simulink library "csc_thm_thermal_system_sim_lib"  (R2014b)
settings: Solver=ode45  StartTime=0.0  StopTime=10.0  RelTol=1e-3
values from neighbouring files (symbols this model uses):
  thm_model_update_counter = round(thm_time_step/sim_time_step_size)    [csc_thm_thermal_system_sim_prep.m]
undefined symbols (not defined in the file or in its folder): stm_time_step
libraries: util_info_lib x1, csc_stm_simplified_temperature_model_collection_lib x1, simulink x1
settings Model: Creator=escrane  LastModifiedBy=mstewart

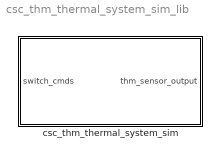
== system csc_thm_thermal_system_sim_lib ==
  csc_thm_thermal_system_sim : Subsystem  SystemSampleTime=stm_time_step

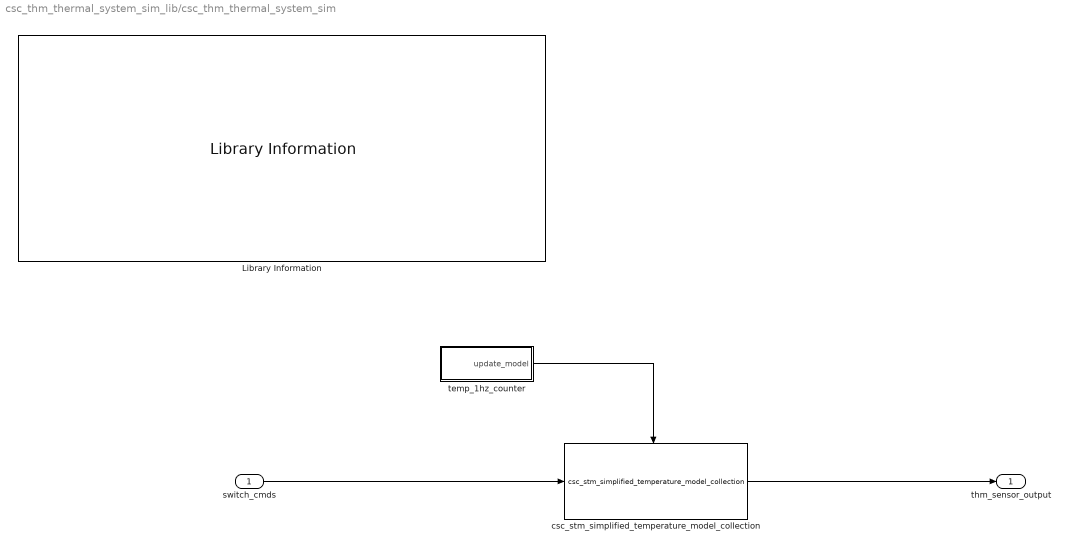
== system csc_thm_thermal_system_sim_lib/csc_thm_thermal_system_sim ==
  switch_cmds : Inport
  Library Information : util_info_lib/Library Information  owner='escrane'
  csc_stm_simplified_temperature_model_collection : csc_stm_simplified_temperature_model_collection_lib/csc_stm_simplified_temperature_model_collection  SystemSampleTime=-1
  temp_1hz_counter : Subsystem  TreatAsAtomicUnit=on
  thm_sensor_output : Outport
  wires:
  csc_stm_simplified_temperature_model_collection/1 -> thm_sensor_output/1
  switch_cmds/1 -> csc_stm_simplified_temperature_model_collection/1
  temp_1hz_counter/1(update_model) -> csc_stm_simplified_temperature_model_collection/Enable

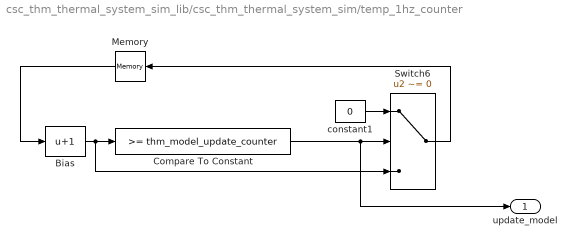
== system csc_thm_thermal_system_sim_lib/csc_thm_thermal_system_sim/temp_1hz_counter ==
  Bias : Bias  Bias=1
  Compare To Constant : simulink/Logic and Bit Operations/Compare To Constant  relop=>=  const=thm_model_update_counter  OutDataTypeStr=uint8
  Memory : Memory  X0=thm_model_update_counter  InheritSampleTime=on
  Switch6 : Switch  Criteria=u2 ~= 0  InputSameDT=on
  constant1 : Constant  Value=0
  update_model : Outport
  wires:
  constant1/1 -> Switch6/1
  Bias/1 -> Compare To Constant/1, Switch6/3
  Compare To Constant/1 -> Switch6/2, update_model/1
  Switch6/1 -> Memory/1
  Memory/1 -> Bias/1
